simulink subsystem "PowertrainState"  (R2023b)
settings: Solver=VariableStepAuto  StartTime=0.0  StopTime=10.0  RelTol=1e-3
settings Model: DataDictionary=Contactors_data.sldd  EnableAccessToBaseWorkspace=off  Creator=Elio  LastModifiedBy=Elio

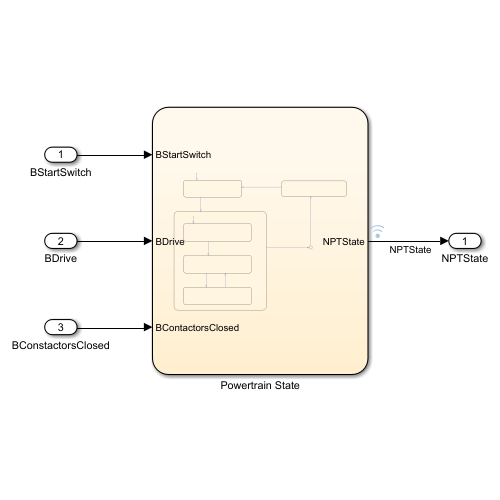
[thumbnail: Simulink's stored preview of the top-level diagram]
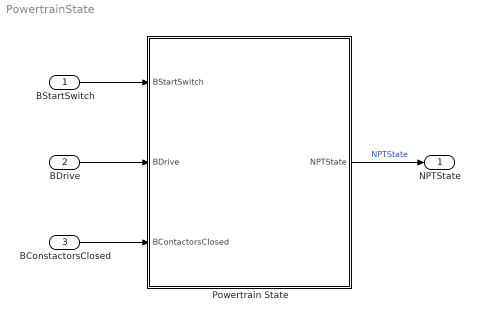
== system PowertrainState ==
  BStartSwitch : Inport
  BDrive : Inport  Port=2
  BConstactorsClosed : Inport  Port=3
  Powertrain State : Stateflow chart  TreatAsAtomicUnit=on
  NPTState : Outport
  wires:
  Powertrain State/1(NPTState) -> NPTState/1  "NPTState"
  BStartSwitch/1 -> Powertrain State/1(BStartSwitch)
  BDrive/1 -> Powertrain State/2(BDrive)
  BConstactorsClosed/1 -> Powertrain State/3(BContactorsClosed)

== stateflow chart PowertrainState/Powertrain State ==
  state OFF
    NPTState = eNPTState.Off;
  state CONTACTORS_OPEN_REQUEST
    NPTState = eNPTState.ContactorsOpenRequest;
  state ON
    state CONTACTORS_CLOSE_REQUEST
      NPTState = eNPTState.ContactorsCloseRequest;
    state CONTACTORS_CLOSED
      NPTState = eNPTState.ContactorsClosed;
    state TORQUE_CONTROL
      NPTState = eNPTState.TorqueControl;
    (default) -> CONTACTORS_CLOSE_REQUEST
    CONTACTORS_CLOSE_REQUEST -> CONTACTORS_CLOSED : [BContactorsClosed]
    CONTACTORS_CLOSED -> TORQUE_CONTROL : [BDrive]
    TORQUE_CONTROL -> CONTACTORS_CLOSED : [!BDrive]
  (default) -> OFF
  CONTACTORS_OPEN_REQUEST -> OFF : [!BContactorsClosed]
  (junction 34) -> CONTACTORS_OPEN_REQUEST
  OFF -> ON : [BStartSwitch]
  ON -> (junction 34) : [!BStartSwitch]
  data: BStartSwitch input; NPTState output double; BDrive input; BContactorsClosed input double
